simulink model "SIM_SAD_DEMO"  (R2025b)
settings: Solver=ode5  StartTime=0.0  StopTime=2*T  FixedStep=0.1  RelTol=1e-3
model workspace (MAT data in the model file):
  Pnull : Simulink.Parameter (value not decoded)
  rho_albedo_medio : Simulink.Parameter (value not decoded)
values from neighbouring files (symbols this model uses):
  Aree = zeros(10,1)    [SCRIPT_SAD_DEMO.m]
  base_seed = base_seed_MC + k    [SCRIPT_SAD_DEMO.m]
  c = astroConstants(5)*1e3    [SCRIPT_SAD_DEMO.m]
  draan = 1.99096871e-7    (= 1.99096871e-07)    [SCRIPT_SAD_DEMO.m]
  dwell_time = 30    [SCRIPT_SAD_DEMO.m]
  eps_att = deg2rad(0.2)    [SCRIPT_SAD_DEMO.m]
  eps_E = deg2rad(astroConstants(63))    [SCRIPT_SAD_DEMO.m]
  eps_h_r = 0.001    [SCRIPT_SAD_DEMO.m]
  eps_w = deg2rad(0.1)    [SCRIPT_SAD_DEMO.m]
  err_max = deg2rad(15)    [SCRIPT_SAD_DEMO.m]
  F_e = 1358    [SCRIPT_SAD_DEMO.m]
  h_r_max = 0.05    [SCRIPT_SAD_DEMO.m]
  h_r_safe = 0.001    [SCRIPT_SAD_DEMO.m]
  j_B = [0.01; 0.05; 0.01]    [SCRIPT_SAD_DEMO.m]
  J_depl = J_nom    [SCRIPT_SAD_DEMO.m]
  JD0 = juliandate(startTime)    [SCRIPT_SAD_DEMO.m]
  k_b = 200000    [SCRIPT_SAD_DEMO.m]
  Kd = K(:, 1:3)    [SCRIPT_SAD_DEMO.m]
  kep = [a,e,incl,raan,w,theta]    [SCRIPT_SAD_DEMO.m]
  Kp = K(:, 4:6)    [SCRIPT_SAD_DEMO.m]
  mu = astroConstants(13)    [SCRIPT_SAD_DEMO.m]
  n = sqrt( (mu/ (a)^3))    [SCRIPT_SAD_DEMO.m]
  n_sun = 2*pi/T_sun    (= 1.99238499086e-07)    [SCRIPT_SAD_DEMO.m]
  Nmat = [ ... (first row only)    [SCRIPT_SAD_DEMO.m]
  r_sun = 1*AU    [SCRIPT_SAD_DEMO.m]
  Re = astroConstants(23)    [SCRIPT_SAD_DEMO.m]
  rf = [ ... (first row only)    [SCRIPT_SAD_DEMO.m]
  rhod = 0.1*ones(10,1)    [SCRIPT_SAD_DEMO.m]
  rhos = zeros(10,1)    [SCRIPT_SAD_DEMO.m]
  SRP = SRP_nom    [SCRIPT_SAD_DEMO.m]
  theta = 0    [SCRIPT_SAD_DEMO.m]
  w0 = w0_nom    [SCRIPT_SAD_DEMO.m]
  w_enter = Control.w_tumbling    [SCRIPT_SAD_DEMO.m]
  w_enter_2 = Control.w_pointing    [SCRIPT_SAD_DEMO.m]
  w_exit = deg2rad(4)    [SCRIPT_SAD_DEMO.m]
  w_exit_2 = deg2rad(1.5)    [SCRIPT_SAD_DEMO.m]
symbols that are objects in the model workspace (value not decoded): Pnull, rho_albedo_medio
undefined symbols (not defined in the file or in its folder): DiscIntNeverNeededParam, Filter, Gyro, Magmeter, MTQ, q, RW, Sun_sensor
libraries: matrix_library x41, LIBRARY_SAD x40, simulink x1, cstblocks x1
(part 2 of 4)

== system SIM_SAD_DEMO/Subsystem ==
  q_e : Inport
  Constant : Constant  Value=0
  Constant1 : Constant
  Demux : Demux
  Gain : Gain  Gain=2
  Gain1 : Gain  Gain=2
  Gain2 : Gain  Gain=2
  Gain3 : Gain  Gain=-1
  Product : Product
  Relational Operator : RelationalOperator  Operator=<=  OutDataTypeStr=boolean  RndMeth=Simplest  InputSameDT=off
  Switch : Switch  Criteria=u2 > Threshold  SaturateOnIntegerOverflow=off  InputSameDT=off
  Vector Concatenate : Concatenate  NumInputs=3
  Out1 : Outport
  wires:
  Vector Concatenate/1 -> Product/1
  Demux/3 -> Gain2/1
  Gain3/1 -> Switch/3
  Gain2/1 -> Vector Concatenate/3
  Constant/1 -> Relational Operator/2
  Relational Operator/1 -> Switch/2
  Constant1/1 -> Switch/1, Gain3/1
  Gain1/1 -> Vector Concatenate/2
  Demux/4 -> Relational Operator/1
  Switch/1 -> Product/2
  Demux/1 -> Gain/1
  Demux/2 -> Gain1/1
  Gain/1 -> Vector Concatenate/1
  Product/1 -> Out1/1
  q_e/1 -> Demux/1

== system SIM_SAD_DEMO/q-->DCM ==
  note: ORTHONORMALITY ERROR A_B/N RECONSTRUCTED CHECK
  q_e : Inport
  Demux1 : Demux  Outputs=9
  Demux2 : Demux
  Display : Display
  Gain4 : Gain  Gain=2
  Gain5 : Gain  Gain=2
  I : Constant  Value=[1,0,0;0,1,0;0,0,1]
  I1 : Constant  Value=[1,0,0;0,1,0;0,0,1]
  MatrixMultiply : Product  Multiplication=Matrix(*)
  MatrixMultiply1 : Product  Multiplication=Matrix(*)
  MatrixMultiply2 : Product  Multiplication=Matrix(*)
  Product1 : Product
  Product2 : Product
  Reshape1 : Reshape  OutputDimensionality=Customize  OutputDimensions=[9,1]
  Scope1 : Scope  NumInputPorts=9
      settings: ActiveDisplayYMinimum=0.78091180257448345  ActiveDisplayYMaximum=1.0243231881597876  DataLoggingVariableName=ScopeData56
  Square : Math  Operator=square
  Sum4 : Sum  Inputs=+-
  Sum5 : Sum  Inputs=+-
  Sum6 : Sum  Inputs=-++
  To Workspace2 : ToWorkspace  VariableName=A_e  SampleTime=-1
  Transpose : Math  Operator=transpose
  Transpose2 : Math  Operator=transpose
  Vector Concatenate1 : Concatenate  NumInputs=3
  "[qΛ]" : Subsystem
  A_B/N_e : Outport
  wires:
  Demux1/2 -> Scope1/2  "A_12"
  MatrixMultiply/1 -> Sum4/2  "qTq"
  Demux2/3 -> Vector Concatenate1/3
  Gain5/1 -> Product1/2  "2q4"
  Product1/1 -> Sum6/1  "2*q4*[qΛ ]"
  Demux2/4 -> Gain5/1, Square/1  "q4"
  Demux1/6 -> Scope1/6  "A_23"
  Product2/1 -> Sum6/2  "(q4^2-qTq)*I"
  Demux2/1 -> Vector Concatenate1/1
  Gain4/1 -> Sum6/3  "2*q*qT"
  Demux1/5 -> Scope1/5  "A_22"
  I1/1 -> Sum5/2
  "[qΛ]"/1("[qΛ]") -> Product1/1
  MatrixMultiply1/1 -> Gain4/1  "qqT"
  Transpose2/1 -> MatrixMultiply2/1  "qT"
  Square/1 -> Sum4/1
  Demux1/8 -> Scope1/8  "A_32"
  Sum4/1 -> Product2/1
  Demux1/7 -> Scope1/7  "A_31"
  I/1 -> Product2/2
  Demux1/9 -> Scope1/9  "A_33"
  Vector Concatenate1/1 -> Transpose/1, MatrixMultiply1/1, MatrixMultiply/2  "q"
  Demux2/2 -> Vector Concatenate1/2
  Sum6/1 -> Transpose2/1, MatrixMultiply2/2, Reshape1/1, To Workspace2/1, A_B/N_e/1  "A_B/N"
  Demux1/1 -> Scope1/1  "A_11"
  MatrixMultiply2/1 -> Sum5/1  "qTq"
  Demux1/4 -> Scope1/4  "A_21"
  Transpose/1 -> MatrixMultiply1/2, MatrixMultiply/1  "qT"
  Reshape1/1 -> Demux1/1
  q_e/1 -> Demux2/1, "[qΛ]"/1(q), Display/1
  Demux1/3 -> Scope1/3  "A_13"

== system SIM_SAD_DEMO/q-->DCM1 ==
  note: ORTHONORMALITY ERROR A_B/N RECONSTRUCTED CHECK
  q_m : Inport
  Demux1 : Demux  Outputs=9
  Demux2 : Demux
  Display : Display
  Gain4 : Gain  Gain=2
  Gain5 : Gain  Gain=2
  I : Constant  Value=[1,0,0;0,1,0;0,0,1]
  I1 : Constant  Value=[1,0,0;0,1,0;0,0,1]
  MatrixMultiply : Product  Multiplication=Matrix(*)
  MatrixMultiply1 : Product  Multiplication=Matrix(*)
  MatrixMultiply2 : Product  Multiplication=Matrix(*)
  Product1 : Product
  Product2 : Product
  Reshape1 : Reshape  OutputDimensionality=Customize  OutputDimensions=[9,1]
  Scope1 : Scope  NumInputPorts=9
      settings: ActiveDisplayYMinimum=0.78091180257448345  ActiveDisplayYMaximum=1.0243231881597876  DataLoggingVariableName=ScopeData56
  Square : Math  Operator=square
  Sum4 : Sum  Inputs=+-
  Sum5 : Sum  Inputs=+-
  Sum6 : Sum  Inputs=-++
  Transpose : Math  Operator=transpose
  Transpose2 : Math  Operator=transpose
  Vector Concatenate1 : Concatenate  NumInputs=3
  "[qΛ]" : Subsystem
  A_B/N_m : Outport
  wires:
  Demux1/2 -> Scope1/2  "A_12"
  MatrixMultiply/1 -> Sum4/2  "qTq"
  Demux2/3 -> Vector Concatenate1/3
  Gain5/1 -> Product1/2  "2q4"
  Product1/1 -> Sum6/1  "2*q4*[qΛ ]"
  Demux2/4 -> Gain5/1, Square/1  "q4"
  Demux1/6 -> Scope1/6  "A_23"
  Product2/1 -> Sum6/2  "(q4^2-qTq)*I"
  Demux2/1 -> Vector Concatenate1/1
  Gain4/1 -> Sum6/3  "2*q*qT"
  Demux1/5 -> Scope1/5  "A_22"
  I1/1 -> Sum5/2
  "[qΛ]"/1("[qΛ]") -> Product1/1
  MatrixMultiply1/1 -> Gain4/1  "qqT"
  Transpose2/1 -> MatrixMultiply2/1  "qT"
  Square/1 -> Sum4/1
  Demux1/8 -> Scope1/8  "A_32"
  Sum4/1 -> Product2/1
  Demux1/7 -> Scope1/7  "A_31"
  I/1 -> Product2/2
  Demux1/9 -> Scope1/9  "A_33"
  Vector Concatenate1/1 -> Transpose/1, MatrixMultiply1/1, MatrixMultiply/2  "q"
  Demux2/2 -> Vector Concatenate1/2
  Sum6/1 -> Transpose2/1, MatrixMultiply2/2, Reshape1/1, A_B/N_m/1  "A_B/N"
  Demux1/1 -> Scope1/1  "A_11"
  MatrixMultiply2/1 -> Sum5/1  "qTq"
  Demux1/4 -> Scope1/4  "A_21"
  Transpose/1 -> MatrixMultiply1/2, MatrixMultiply/1  "qT"
  Reshape1/1 -> Demux1/1
  q_m/1 -> Demux2/1, "[qΛ]"/1(q), Display/1
  Demux1/3 -> Scope1/3  "A_13"

== system SIM_SAD_DEMO/ACTUATORS/Detumbling (MTQ only) ==
  note: REACTION WHEEL
  note: MAGNETORQUERS
  M_c : Inport
  B_B_m : Inport  Port=2
  h_r_feed : Inport  Port=3
  Constant : Constant  Value=0
  Constant1 : Constant  Value=RW.A
  Cross Product : matrix_library/Cross Product
  Cross Product2 : matrix_library/Cross Product
  Delay : Delay  DelayLength=1  SampleTime=q.Ts
  Demux : Demux  Outputs=3
  Discrete-Time Integrator : DiscreteIntegrator  InitialConditionSource=external  SampleTime=-1  ICPrevOutput=DiscIntNeverNeededParam  ICPrevScaledInput=DiscIntNeverNeededParam
  Divide : Product  Inputs=*/
  MatrixMultiply : Product  Multiplication=Matrix(*)
  Norm1 : Subsystem
  Saturation3 : Saturate  UpperLimit=MTQ.D_max_XY  LowerLimit=-MTQ.D_max_XY
  Saturation4 : Saturate  UpperLimit=MTQ.D_max_XY  LowerLimit=-MTQ.D_max_XY
  Saturation5 : Saturate  UpperLimit=MTQ.D_max_Z  LowerLimit=-MTQ.D_max_Z
  Scope : Scope
      settings: ActiveDisplayYMinimum=-14.411553950631344  ActiveDisplayYMaximum=16.201380468990443  DataLoggingVariableName=ScopeData111
  Scope6 : Scope
      settings: ActiveDisplayYMinimum=-2.5  ActiveDisplayYMaximum=2.5  DataLoggingVariableName=ScopeData112
  Square1 : Math  Operator=square
  Sum : Sum
  Vector Concatenate1 : Concatenate  NumInputs=3
  M_act : Outport
  h_r : Outport  Port=2
  wires:
  Cross Product2/1 -> Sum/1  "M_MTQ"
  Saturation3/1 -> Vector Concatenate1/1
  Demux/2 -> Saturation4/1
  Demux/1 -> Saturation3/1
  Saturation4/1 -> Vector Concatenate1/2
  Norm1/1(Out1) -> Square1/1
  Cross Product/1 -> Divide/1
  Square1/1 -> Divide/2
  Saturation5/1 -> Vector Concatenate1/3
  Vector Concatenate1/1 -> Cross Product2/1, Scope6/1  "D_eff"
  Divide/1 -> Scope/1, Demux/1  "D"
  Demux/3 -> Saturation5/1
  B_B_m/1 -> Cross Product2/2, Cross Product/1, Norm1/1(In1)  "B_B_m"
  M_c/1 -> Cross Product/2
  Constant/1 -> MatrixMultiply/2, Discrete-Time Integrator/1  "h_r_dot"
  Discrete-Time Integrator/1 -> h_r/1  "h_r"
  h_r_feed/1 -> Delay/1
  Sum/1 -> M_act/1
  Constant1/1 -> MatrixMultiply/1
  MatrixMultiply/1 -> Sum/2  "M_RW"
  Delay/1 -> Discrete-Time Integrator/2

== system SIM_SAD_DEMO/ACTUATORS/Norm ==
  note: square
  B_B_m : Inport
  Sqrt : Sqrt
  Square1 : Math  Operator=square
  Sum of Elements : Sum  Inputs=+
  Out1 : Outport
  wires:
  Sum of Elements/1 -> Sqrt/1
  B_B_m/1 -> Square1/1
  Sqrt/1 -> Out1/1
  Square1/1 -> Sum of Elements/1

== system SIM_SAD_DEMO/ACTUATORS/Norm1 ==
  note: square
  In1 : Inport
  Sqrt : Sqrt
  Square1 : Math  Operator=square
  Sum of Elements : Sum  Inputs=+
  Out1 : Outport
  wires:
  Sum of Elements/1 -> Sqrt/1
  In1/1 -> Square1/1
  Sqrt/1 -> Out1/1
  Square1/1 -> Sum of Elements/1

== system SIM_SAD_DEMO/ACTUATORS/RW Desaturation ==
  note: MAGNETORQUERS
  note: REACTION WHEEL (only for h_r)
  h_r_feed : Inport
  B_B_m : Inport  Port=2
  -M_max : Gain  Gain=-RW.T_max
  Constant : Constant  Value=RW.A
  Cross Product : matrix_library/Cross Product
  Delay : Delay  DelayLength=1  SampleTime=q.Ts
  Demux : Demux  Outputs=3
  Discrete-Time Integrator : DiscreteIntegrator  InitialConditionSource=external  SampleTime=-1  ICPrevOutput=DiscIntNeverNeededParam  ICPrevScaledInput=DiscIntNeverNeededParam
  Divide : Product  Inputs=*/
  M_max : Gain  Gain=RW.T_max
  MatrixMultiply : Product  Multiplication=Matrix(*)
  Saturation3 : Saturate  UpperLimit=MTQ.D_max_XY  LowerLimit=-MTQ.D_max_XY
  Saturation4 : Saturate  UpperLimit=MTQ.D_max_XY  LowerLimit=-MTQ.D_max_XY
  Saturation5 : Saturate  UpperLimit=MTQ.D_max_Z  LowerLimit=-MTQ.D_max_Z
  Scope{,1..6} (7 alike) : Scope
      Scope settings: ActiveDisplayYMinimum=-1  ActiveDisplayYMaximum=1  DataLoggingVariableName=ScopeData120
      Scope1 settings: ActiveDisplayYMinimum=-1  ActiveDisplayYMaximum=1  DataLoggingVariableName=ScopeData122
      Scope2 settings: ActiveDisplayYMinimum=-1  ActiveDisplayYMaximum=1  DataLoggingVariableName=ScopeData123
      Scope3 settings: ActiveDisplayYMinimum=-1  ActiveDisplayYMaximum=1  DataLoggingVariableName=ScopeData124
      Scope4 settings: ActiveDisplayYMinimum=-1  ActiveDisplayYMaximum=1  DataLoggingVariableName=ScopeData126
      Scope5 settings: ActiveDisplayYMinimum=-1  ActiveDisplayYMaximum=1  DataLoggingVariableName=ScopeData127
      Scope6 settings: ActiveDisplayYMinimum=-0.0068500524485620249  ActiveDisplayYMaximum=0.056316672494284674  DataLoggingVariableName=ScopeData128
  Sign : Signum
  Sign1 : Signum
  Square : Math  Operator=square
  Vector Concatenate1 : Concatenate  NumInputs=3
  vector_norm1 : LIBRARY_SAD/vector_norm  SystemSampleTime=-1  VariantActivationTime=update diagram  EmptyChoice=off  PassThrough=off  PassThroughVariantControl=(default)  EmptyChoiceVariantControl=(default)  AllowFlexibleInterface=on  Latency=0  AutoFrameSizeCalculation=off
  M_act : Outport
  h_r : Outport  Port=2
  wires:
  h_r_feed/1 -> Delay/1
  Delay/1 -> Scope6/1, Discrete-Time Integrator/2
  Sign/1 -> -M_max/1
  Discrete-Time Integrator/1 -> Sign/1, Sign1/1, Scope1/1, h_r/1  "h_r"
  B_B_m/1 -> Scope4/1, Cross Product/2, vector_norm1/1
  Sign1/1 -> M_max/1
  vector_norm1/1 -> Square/1
  M_max/1 -> MatrixMultiply/2
  Square/1 -> Divide/2
  Demux/1 -> Saturation3/1
  Divide/1 -> Demux/1  "D"
  Demux/3 -> Saturation5/1
  Saturation5/1 -> Vector Concatenate1/3
  Saturation3/1 -> Vector Concatenate1/1
  Demux/2 -> Saturation4/1
  Saturation4/1 -> Vector Concatenate1/2
  Vector Concatenate1/1 -> Cross Product/1, Scope/1  "D_eff"
  Cross Product/1 -> M_act/1, Scope3/1  "M_MTQ_desat"
  -M_max/1 -> Discrete-Time Integrator/1, Scope2/1  "T_RW=h_r_dot"
  MatrixMultiply/1 -> Scope5/1, Divide/1
  Constant/1 -> MatrixMultiply/1

== system SIM_SAD_DEMO/ACTUATORS/Slew//tracking (MTQ + RW) ==
  note: MAGNETORQUERS
  note: REACTION WHEEL
  M_c : Inport
  B_B_m : Inport  Port=2
  w_est : Inport  Port=3
  h_r_feed : Inport  Port=4
  A* (pseudo-inverse) : Subsystem
  Constant : Constant  Value=RW.A
  Constant1 : Constant  Value=RW.A
  Cross Product : matrix_library/Cross Product
  Cross Product1 : matrix_library/Cross Product
  Cross Product2 : matrix_library/Cross Product
  Delay : Delay  DelayLength=1  SampleTime=q.Ts
  Demux : Demux  Outputs=3
  Divide : Product  Inputs=*/
  Gain : Gain  Gain=-1
  Gain1 : Gain  Gain=-1
  Integrator : Integrator  InitialConditionSource=external
  MatrixMultiply : Product  Multiplication=Matrix(*)
  MatrixMultiply1 : Product  Multiplication=Matrix(*)
  MatrixMultiply2 : Product  Multiplication=Matrix(*)
  Norm1 : Subsystem
  Rate Limiter : RateLimiter  RisingSlewLimit=0.1  FallingSlewLimit=-0.1  SampleTimeMode=inherited
  Saturation : Saturate  UpperLimit=RW.T_max  LowerLimit=-RW.T_max
  Saturation3 : Saturate  UpperLimit=MTQ.D_max_XY  LowerLimit=-MTQ.D_max_XY
  Saturation4 : Saturate  UpperLimit=MTQ.D_max_XY  LowerLimit=-MTQ.D_max_XY
  Saturation5 : Saturate  UpperLimit=MTQ.D_max_Z  LowerLimit=-MTQ.D_max_Z
  Scope{,1..2,6} (4 alike) : Scope
      Scope settings: ActiveDisplayYMinimum=-14.411553950631344  ActiveDisplayYMaximum=16.201380468990443  DataLoggingVariableName=ScopeData113
      Scope1 settings: ActiveDisplayYMinimum=-0.00988821849985589  ActiveDisplayYMaximum=0.00899396649870301  DataLoggingVariableName=ScopeData116
      Scope2 settings: ActiveDisplayYMinimum=-0.000160369873046875  ActiveDisplayYMaximum=0.00015304565429687502  DataLoggingVariableName=ScopeData117
      Scope6 settings: ActiveDisplayYMinimum=-2.5  ActiveDisplayYMaximum=2.5  DataLoggingVariableName=ScopeData118
  Square1 : Math  Operator=square
  Sum : Sum  Inputs=++-
  Sum1 : Sum
  Vector Concatenate1 : Concatenate  NumInputs=3
  M_act : Outport
  h_r : Outport  Port=2
  wires:
  B_B_m/1 -> Norm1/1(In1), Cross Product/1, Cross Product2/2  "B_B_m"
  Square1/1 -> Divide/2
  Demux/1 -> Saturation3/1
  Vector Concatenate1/1 -> Cross Product2/1, Scope6/1  "D_eff"
  Saturation3/1 -> Vector Concatenate1/1
  Saturation5/1 -> Vector Concatenate1/3
  Saturation4/1 -> Vector Concatenate1/2
  Cross Product2/1 -> Sum/3, Scope2/1, Sum1/2  "M_MTQ"
  Cross Product/1 -> Divide/1
  Demux/2 -> Saturation4/1
  Norm1/1(Out1) -> Square1/1
  Demux/3 -> Saturation5/1
  Divide/1 -> Scope/1, Demux/1  "D"
  M_c/1 -> Cross Product/2, Sum/1  "M_c"
  w_est/1 -> Cross Product1/1
  MatrixMultiply/1 -> Cross Product1/2
  Constant/1 -> MatrixMultiply/1
  Cross Product1/1 -> Sum/2
  A* (pseudo-inverse)/1(A*) -> Gain/1
  Gain/1 -> MatrixMultiply1/1
  MatrixMultiply1/1 -> MatrixMultiply2/2, Rate Limiter/1  "h_r_dot"
  Rate Limiter/1 -> Integrator/1  "h_r_dot"
  h_r_feed/1 -> Delay/1
  Delay/1 -> Integrator/2
  Integrator/1 -> h_r/1, MatrixMultiply/2  "h_r"
  Constant1/1 -> MatrixMultiply2/1
  MatrixMultiply2/1 -> Gain1/1
  Gain1/1 -> Saturation/1
  Sum1/1 -> M_act/1
  Saturation/1 -> Scope1/1, Sum1/1  "M_RW"
  Sum/1 -> MatrixMultiply1/2

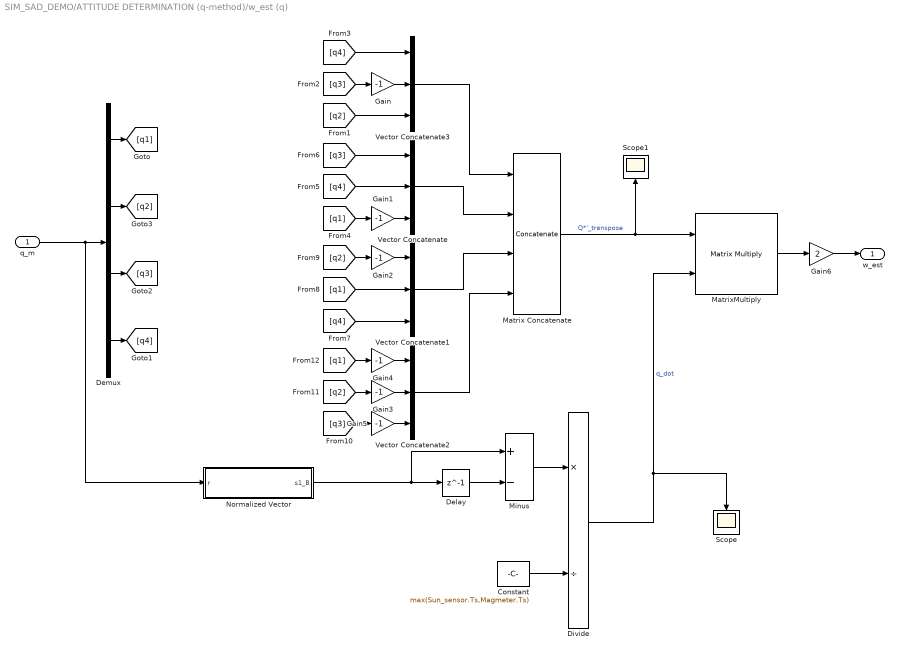
== system SIM_SAD_DEMO/ATTITUDE DETERMINATION (q-method)/w_est (q) ==
  q_m : Inport
  Constant : Constant  Value=max(Sun_sensor.Ts,Magmeter.Ts)
  Delay : Delay  DelayLength=1
  Demux : Demux
  Divide : Product  Inputs=*/
  Gain{,1..5} (6 alike) : Gain  Gain=-1
  Gain6 : Gain  Gain=2
  Matrix Concatenate : Concatenate  NumInputs=4  Mode=Multidimensional array  ConcatenateDimension=2
  MatrixMultiply : Product  Multiplication=Matrix(*)
  Minus : Sum  Inputs=+-
  Normalized Vector : Subsystem
  Scope : Scope
      settings: ActiveDisplayYMinimum=-1  ActiveDisplayYMaximum=1  DataLoggingVariableName=ScopeData67
  Scope1 : Scope
      settings: ActiveDisplayYMinimum=-1  ActiveDisplayYMaximum=1  DataLoggingVariableName=ScopeData68
  Vector Concatenate{,1..3} (4 alike) : Concatenate  NumInputs=3
  w_est : Outport
  wires:
  q_m/1 -> Normalized Vector/1(r), Demux/1
  Demux/1 -> [q1]
  Demux/2 -> [q2]
  Demux/3 -> [q3]
  Demux/4 -> [q4]
  [q4] -> Vector Concatenate3/1
  [q3] -> Gain/1
  Gain/1 -> Vector Concatenate3/2
  [q2] -> Vector Concatenate3/3
  [q1] -> Gain1/1
  [q3] -> Vector Concatenate/1
  [q4] -> Vector Concatenate1/3
  [q2] -> Gain2/1
  [q3] -> Gain5/1
  [q2] -> Gain3/1
  [q1] -> Gain4/1
  Gain3/1 -> Vector Concatenate2/2
  [q1] -> Vector Concatenate1/2
  [q4] -> Vector Concatenate/2
  Gain1/1 -> Vector Concatenate/3
  Gain2/1 -> Vector Concatenate1/1
  Gain4/1 -> Vector Concatenate2/1
  Gain5/1 -> Vector Concatenate2/3
  Vector Concatenate3/1 -> Matrix Concatenate/1
  Vector Concatenate/1 -> Matrix Concatenate/2
  Vector Concatenate1/1 -> Matrix Concatenate/3
  Vector Concatenate2/1 -> Matrix Concatenate/4
  Delay/1 -> Minus/2
  Matrix Concatenate/1 -> MatrixMultiply/1, Scope1/1  "Q*'_transpose"
  MatrixMultiply/1 -> Gain6/1
  Gain6/1 -> w_est/1
  Minus/1 -> Divide/1
  Divide/1 -> Scope/1, MatrixMultiply/2  "q_dot"
  Constant/1 -> Divide/2
  Normalized Vector/1(s1_B) -> Delay/1, Minus/1

== system SIM_SAD_DEMO/ATTITUDE TARGET (Sun Pointing)/Normalized Vector ==
  In1 : Inport
  Divide : Product  Inputs=*/
  vector_norm : LIBRARY_SAD/vector_norm  SystemSampleTime=-1  VariantActivationTime=update diagram  EmptyChoice=off  PassThrough=off  PassThroughVariantControl=(default)  EmptyChoiceVariantControl=(default)  AllowFlexibleInterface=on  Latency=0  AutoFrameSizeCalculation=off
  Out1 : Outport
  wires:
  vector_norm/1 -> Divide/2
  In1/1 -> Divide/1, vector_norm/1
  Divide/1 -> Out1/1

== system SIM_SAD_DEMO/ATTITUDE TARGET (Sun Pointing)/Normalized Vector2 ==
  r : Inport
  Divide : Product  Inputs=*/
  vector_norm : LIBRARY_SAD/vector_norm  SystemSampleTime=-1  VariantActivationTime=update diagram  EmptyChoice=off  PassThrough=off  PassThroughVariantControl=(default)  EmptyChoiceVariantControl=(default)  AllowFlexibleInterface=on  Latency=0  AutoFrameSizeCalculation=off
  s2_B : Outport
  wires:
  Divide/1 -> s2_B/1
  r/1 -> Divide/1, vector_norm/1
  vector_norm/1 -> Divide/2

== system SIM_SAD_DEMO/CONTROL/B_dot (Detumbling) ==
  w_est : Inport
  B_B_m : Inport  Port=2
  Cross Product : matrix_library/Cross Product
  Cross Product1 : matrix_library/Cross Product
  Gain : Gain  Gain=-1
  Gain1 : Gain  Gain=-k_b
  Scope{,1..3} (4 alike) : Scope
      Scope settings: ActiveDisplayYMinimum=-4.1909426960566919E-5  ActiveDisplayYMaximum=6.5793655893850854E-5  DataLoggingVariableName=ScopeData86
      Scope1 settings: ActiveDisplayYMinimum=-1  ActiveDisplayYMaximum=1  DataLoggingVariableName=ScopeData87
      Scope2 settings: ActiveDisplayYMinimum=-1  ActiveDisplayYMaximum=1  DataLoggingVariableName=ScopeData88
      Scope3 settings: ActiveDisplayYMinimum=-1  ActiveDisplayYMaximum=1  DataLoggingVariableName=ScopeData89
  M_c_detumbling : Outport
  wires:
  Cross Product1/1 -> Scope2/1, M_c_detumbling/1  "M_c_detumbling"
  Gain1/1 -> Scope3/1, Cross Product1/1  "D_req"
  Cross Product/1 -> Scope1/1, Gain1/1  "B_dot_m"
  Gain/1 -> Cross Product/1
  B_B_m/1 -> Cross Product/2, Cross Product1/2, Scope/1  "B_B_m"
  w_est/1 -> Gain/1

== system SIM_SAD_DEMO/CONTROL/ERROR VECTOR ==
  A_B/T_e : Inport
  Demux : Demux  Outputs=9
  Display : Display
  Gain : Gain  Gain=0.5
  Gain1 : Gain  Gain=0.5
  Gain2 : Gain  Gain=0.5
  Reshape : Reshape  OutputDimensionality=Customize  OutputDimensions=[9,1]
  Sum : Sum  Inputs=+-
  Sum1 : Sum  Inputs=+-
  Sum2 : Sum  Inputs=+-
  Terminator : Terminator
  Terminator1 : Terminator
  Terminator2 : Terminator
  Vector Concatenate : Concatenate  NumInputs=3
  as : Outport
  wires:
  A_B/T_e/1 -> Reshape/1
  Reshape/1 -> Demux/1
  Demux/1 -> Terminator1/1  "A_11"
  Demux/2 -> Sum2/2  "A_21"
  Demux/3 -> Sum1/1  "A_31"
  Demux/4 -> Sum2/1  "A_12"
  Demux/5 -> Terminator/1  "A_22"
  Demux/6 -> Sum/2  "A_32"
  Demux/7 -> Sum1/2  "A_13"
  Demux/8 -> Sum/1  "A_23"
  Demux/9 -> Terminator2/1  "A_33"
  Sum/1 -> Gain/1
  Sum1/1 -> Gain1/1
  Sum2/1 -> Gain2/1
  Gain/1 -> Vector Concatenate/1  "first  component"
  Gain1/1 -> Vector Concatenate/2  "second component"
  Gain2/1 -> Vector Concatenate/3  "third component"
  Vector Concatenate/1 -> as/1, Display/1

== system SIM_SAD_DEMO/CONTROL/RW Desaturation ==
  Constant : Constant  Value=0
  Constant1 : Constant  Value=0
  Constant2 : Constant  Value=0
  Vector Concatenate : Concatenate  NumInputs=3
  M_c_desat : Outport
  wires:
  Constant/1 -> Vector Concatenate/1
  Constant2/1 -> Vector Concatenate/3
  Constant1/1 -> Vector Concatenate/2
  Vector Concatenate/1 -> M_c_desat/1

== system SIM_SAD_DEMO/CONTROL/Slew Manouvre//pointing ==
  note: CONTROL LOGIC: u = -kp*as - kd*w
      | as = components of matrix A_e
  w_est : Inport
  as : Inport  Port=2
  Constant : Constant  Value=Kd
  Constant1 : Constant  Value=Kp
  Gain : Gain  Gain=-1
  Gain1 : Gain  Gain=-1
  Matrix Multiply : Product  Multiplication=Matrix(*)
  Matrix Multiply1 : Product  Multiplication=Matrix(*)
  Scope : Scope
      settings: ActiveDisplayYMinimum=-0.23306272336823153  ActiveDisplayYMaximum=0.11744428316780303  DataLoggingVariableName=ScopeData90
  Sum of Elements : Sum
  Mc_slew : Outport
  wires:
  Gain/1 -> Matrix Multiply/2
  as/1 -> Gain1/1
  Matrix Multiply/1 -> Sum of Elements/1
  Matrix Multiply1/1 -> Sum of Elements/2
  Constant1/1 -> Matrix Multiply1/1
  w_est/1 -> Gain/1
  Gain1/1 -> Matrix Multiply1/2
  Sum of Elements/1 -> Scope/1, Mc_slew/1
  Constant/1 -> Matrix Multiply/1

== system SIM_SAD_DEMO/CONTROL/Tracking ==
  note: CONTROL LOGIC: u = -kp*alpha - kd*w
      | alpha = [alpha_x; alpha_y; alpha_z] rotations under the hypothesis of small angles
  w_est : Inport
  alpha : Inport  Port=2
  Constant : Constant  Value=Kd
  Constant1 : Constant  Value=Kp
  Gain : Gain  Gain=-1
  Gain1 : Gain  Gain=-1
  Matrix Multiply : Product  Multiplication=Matrix(*)
  Matrix Multiply1 : Product  Multiplication=Matrix(*)
  Scope : Scope
      settings: ActiveDisplayYMinimum=-0.23306272336823153  ActiveDisplayYMaximum=0.11744428316780303  DataLoggingVariableName=ScopeData93
  Sum of Elements : Sum
  Mc_tracking : Outport
  wires:
  Gain1/1 -> Matrix Multiply1/2
  Gain/1 -> Matrix Multiply/2
  Sum of Elements/1 -> Scope/1, Mc_tracking/1
  w_est/1 -> Gain/1
  Matrix Multiply1/1 -> Sum of Elements/2
  Matrix Multiply/1 -> Sum of Elements/1
  Constant1/1 -> Matrix Multiply1/1
  Constant/1 -> Matrix Multiply/1
  alpha/1 -> Gain1/1

== system SIM_SAD_DEMO/DCM ---> q/q-->DCM (CHECK) ==
  note: ORTHONORMALITY ERROR A_B/N RECONSTRUCTED CHECK
  q_norm : Inport
  Demux1 : Demux  Outputs=9
  Demux2 : Demux
  Display : Display
  Gain4 : Gain  Gain=2
  Gain5 : Gain  Gain=2
  I : Constant  Value=[1,0,0;0,1,0;0,0,1]
  I1 : Constant  Value=[1,0,0;0,1,0;0,0,1]
  MatrixMultiply : Product  Multiplication=Matrix(*)
  MatrixMultiply1 : Product  Multiplication=Matrix(*)
  MatrixMultiply2 : Product  Multiplication=Matrix(*)
  Product1 : Product
  Product2 : Product
  Reshape1 : Reshape  OutputDimensionality=Customize  OutputDimensions=[9,1]
  Scope : Scope
      settings: ActiveDisplayYMinimum=-1  ActiveDisplayYMaximum=1  DataLoggingVariableName=ScopeData57
  Scope1 : Scope  NumInputPorts=9
      settings: ActiveDisplayYMinimum=-1.2499999988864972  ActiveDisplayYMaximum=1.2499999998762776  DataLoggingVariableName=ScopeData56
  Square : Math  Operator=square
  Sum4 : Sum  Inputs=+-
  Sum5 : Sum  Inputs=+-
  Sum6 : Sum  Inputs=-++
  Transpose : Math  Operator=transpose
  Transpose2 : Math  Operator=transpose
  Vector Concatenate1 : Concatenate  NumInputs=3
  "[qΛ]" : Subsystem
  wires:
  Demux1/3 -> Scope1/3  "A_13"
  q_norm/1 -> Display/1, "[qΛ]"/1(q), Demux2/1
  Reshape1/1 -> Demux1/1
  Transpose/1 -> MatrixMultiply/1, MatrixMultiply1/2  "qT"
  Demux1/4 -> Scope1/4  "A_21"
  MatrixMultiply2/1 -> Sum5/1  "qTq"
  Demux1/1 -> Scope1/1  "A_11"
  Sum6/1 -> Reshape1/1, MatrixMultiply2/2, Transpose2/1  "A_B/N"
  Demux2/2 -> Vector Concatenate1/2
  Vector Concatenate1/1 -> MatrixMultiply/2, MatrixMultiply1/1, Transpose/1  "q"
  Demux1/9 -> Scope1/9  "A_33"
  Sum5/1 -> Scope/1
  I/1 -> Product2/2
  Demux1/7 -> Scope1/7  "A_31"
  Sum4/1 -> Product2/1
  Demux1/8 -> Scope1/8  "A_32"
  Square/1 -> Sum4/1
  Transpose2/1 -> MatrixMultiply2/1  "qT"
  MatrixMultiply1/1 -> Gain4/1  "qqT"
  "[qΛ]"/1("[qΛ]") -> Product1/1
  I1/1 -> Sum5/2
  Demux1/5 -> Scope1/5  "A_22"
  Gain4/1 -> Sum6/3  "2*q*qT"
  Demux2/1 -> Vector Concatenate1/1
  Product2/1 -> Sum6/2  "(q4^2-qTq)*I"
  Demux1/6 -> Scope1/6  "A_23"
  Demux2/4 -> Square/1, Gain5/1  "q4"
  Product1/1 -> Sum6/1  "2*q4*[qΛ ]"
  Gain5/1 -> Product1/2  "2q4"
  Demux2/3 -> Vector Concatenate1/3
  MatrixMultiply/1 -> Sum4/2  "qTq"
  Demux1/2 -> Scope1/2  "A_12"

== system SIM_SAD_DEMO/DCM ---> q/vector_norm ==
  r : Inport
  Sqrt : Sqrt
  Square : Math  Operator=square
  Sum of Elements : Sum  Inputs=+
  r_norm : Outport
  wires:
  Sqrt/1 -> r_norm/1
  r/1 -> Square/1
  Sum of Elements/1 -> Sqrt/1
  Square/1 -> Sum of Elements/1

== system SIM_SAD_DEMO/DCM->q (Shepperd Algorithm)/Normalized Vector1 ==
  r : Inport
  Constant : Constant  Value=1e-12
  Divide : Product  Inputs=*/
  Max : MinMax  Function=max  Inputs=2
  vector_norm : LIBRARY_SAD/vector_norm  SystemSampleTime=-1  VariantActivationTime=update diagram  EmptyChoice=off  PassThrough=off  PassThroughVariantControl=(default)  EmptyChoiceVariantControl=(default)  AllowFlexibleInterface=on  Latency=0  AutoFrameSizeCalculation=off
  r_norm : Outport
  wires:
  vector_norm/1 -> Max/1
  r/1 -> Divide/1, vector_norm/1
  Divide/1 -> r_norm/1
  Constant/1 -> Max/2
  Max/1 -> Divide/2

== system SIM_SAD_DEMO/DKE/ALBEDO_TORQUE ==
  note: Solar Radiation Pression Torque
  note: creo un blocco for each che mi permette di eseguire passo a passo ogni singola operazione del prodotto vettoriale, andando poi a crearmi il vettore uscita finale. In input ho un 10x3, però dentro il for each lavoro con delle 3x1 per semplicità, con vettori colonna quindi
  note: scarto i valori negativi perchè significa che mi trovo dalla parte opposta della faccia colpita dal sole, quindi non genero albedo, in quel caso tutto il satellite non viene colpito, quindi non mi serve creare una mask, ma basta semplicemente considerare il vettore nullo
  sun direction inertial : Inport
  Ab_n : Inport  Port=2
  S/C direction : Inport  Port=3
  Constant : Constant  Value=0
  Constant16 : Constant  Value=rf
  Constant2 : Constant  Value=Pnull
  Dot Product : DotProduct  OutDataTypeStr=Inherit: Inherit via internal rule
  For Each Subsystem1 : Subsystem  TreatAsAtomicUnit=on
  Matrix Multiply4 : Product  Multiplication=Matrix(*)
  Max : MinMax  Function=max  Inputs=2
  Normalization : Subsystem
  "Normalization " : Subsystem
  Normalization1 : Subsystem
  Reshape2 : Reshape  OutputDimensionality=Customize  OutputDimensions=[10 3]
  Ricavo i vettori forza1 : Subsystem
  Scope10 : Scope
      settings: ActiveDisplayYMinimum=-8805.2567998384475  ActiveDisplayYMaximum=8127.929464306656  DataLoggingVariableName=ScopeData17
  Scope9 : Scope
      settings: ActiveDisplayYMinimum=-9.2718061255302776E-25  ActiveDisplayYMaximum=2.6543612251060555E-24  DataLoggingVariableName=ScopeData25
  Sum of Elements2 : Sum  Inputs=+  CollapseMode=Specified dimension
  Switch : Switch  Criteria=u2 > Threshold  SaturateOnIntegerOverflow=off  InputSameDT=off
  To Workspace : ToWorkspace  VariableName=AlbRtorque  SampleTime=-1
  Transpose : Math  Operator=transpose
  Albedo_torque : Outport
  wires:
  Sum of Elements2/1 -> Transpose/1, To Workspace/1, Scope9/1
  Matrix Multiply4/1 -> Ricavo i vettori forza1/3(R_B), Normalization/1(In1)
  Normalization1/1(Out1) -> Dot Product/2
  Ricavo i vettori forza1/1(Out1) -> For Each Subsystem1/2(In2)
  For Each Subsystem1/1(Out1) -> Reshape2/1
  S/C direction/1 -> Scope10/1, Matrix Multiply4/2, Normalization1/1(R_N)
  "Normalization "/1(Out1) -> Dot Product/1
  Constant16/1 -> For Each Subsystem1/1(In1)
  Normalization/1(Out1) -> Ricavo i vettori forza1/1(" R_ B direction normalized")
  Dot Product/1 -> Max/1  "Illuminated"
  Ab_n/1 -> Matrix Multiply4/1
  sun direction inertial/1 -> "Normalization "/1(In1)
  Constant2/1 -> Switch/3
  Reshape2/1 -> Sum of Elements2/1
  Constant/1 -> Max/2
  Transpose/1 -> Switch/1
  Switch/1 -> Albedo_torque/1
  Max/1 -> Ricavo i vettori forza1/2(In2), [Illum]  "Illuminated"
  [Illum] -> Switch/2

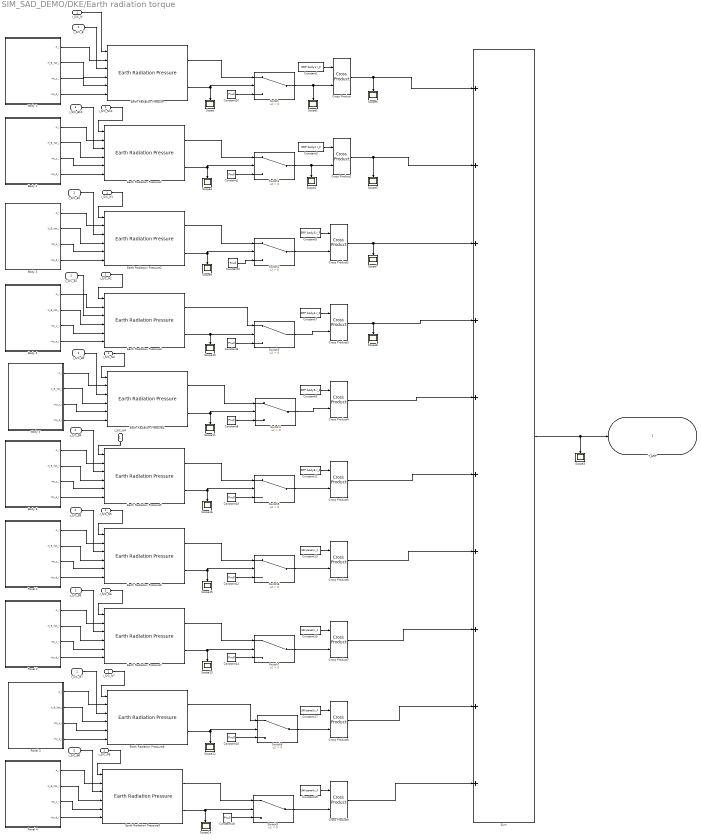
== system SIM_SAD_DEMO/DKE/Earth radiation torque ==
  r_S/C_N : Inport
  r_S/C_B : Inport  Port=2
  Body 1 : Subsystem
  Body 2 : Subsystem
  Body 3 : Subsystem
  Body 4 : Subsystem
  Body 5 : Subsystem
  Body 6 : Subsystem
  Constant1 : Constant  Value=SRP.body1.r_F
  Constant{2,4,6,8,10,12,14,16,18,20} (10 alike) : Constant  Value=Pnull
  Constant11 : Constant  Value=SRP.body6.r_F
  Constant13 : Constant  Value=SRP.panel1.r_F
  Constant15 : Constant  Value=SRP.panel2.r_F
  Constant17 : Constant  Value=SRP.panel3.r_F
  Constant19 : Constant  Value=SRP.panel4.r_F
  Constant3 : Constant  Value=SRP.body2.r_F
  Constant5 : Constant  Value=SRP.body3.r_F
  Constant7 : Constant  Value=SRP.body4.r_F
  Constant9 : Constant  Value=SRP.body5.r_F
  Cross Product{,1..9} (10 alike) : matrix_library/Cross Product
  Earth Radiation Pressure{,1..9} (10 alike) : LIBRARY_SAD/Earth Radiation Pressure  SystemSampleTime=-1  VariantActivationTime=update diagram  EmptyChoice=off  PassThrough=off  PassThroughVariantControl=(default)  EmptyChoiceVariantControl=(default)  AllowFlexibleInterface=on  Latency=0  AutoFrameSizeCalculation=off
  Panel 1 : Subsystem
  Panel 2 : Subsystem
  Panel 3 : Subsystem
  Panel 4 : Subsystem
  Scope{,1..16} (17 alike) : Scope
      Scope settings: ActiveDisplayYMinimum=-1  ActiveDisplayYMaximum=1  DataLoggingVariableName=ScopeData28
      Scope1 settings: ActiveDisplayYMinimum=-1  ActiveDisplayYMaximum=1  DataLoggingVariableName=ScopeData29
      Scope10 settings: DataLoggingVariableName=ScopeData11
      Scope11 settings: DataLoggingVariableName=ScopeData12
      Scope12 settings: DataLoggingVariableName=ScopeData13
      Scope13 settings: DataLoggingVariableName=ScopeData14
      Scope14 settings: DataLoggingVariableName=ScopeData15
      Scope15 settings: DataLoggingVariableName=ScopeData17
      Scope16 settings: DataLoggingVariableName=ScopeData18
      Scope2 settings: ActiveDisplayYMinimum=-1  ActiveDisplayYMaximum=1  DataLoggingVariableName=ScopeData30
      Scope3 settings: ActiveDisplayYMinimum=-5.1359030627651383E-25  ActiveDisplayYMaximum=9.2718061255302776E-25  DataLoggingVariableName=ScopeData31
      Scope4 settings: ActiveDisplayYMinimum=-1  ActiveDisplayYMaximum=1  DataLoggingVariableName=ScopeData32
      Scope5 settings: ActiveDisplayYMinimum=-1  ActiveDisplayYMaximum=1  DataLoggingVariableName=ScopeData33
      Scope6 settings: ActiveDisplayYMinimum=-1  ActiveDisplayYMaximum=1  DataLoggingVariableName=ScopeData34
      Scope7 settings: ActiveDisplayYMinimum=-1  ActiveDisplayYMaximum=1  DataLoggingVariableName=ScopeData35
      Scope8 settings: ActiveDisplayYMinimum=-1  ActiveDisplayYMaximum=1  DataLoggingVariableName=ScopeData36
      Scope9 settings: DataLoggingVariableName=ScopeData10
  Sum : Sum  Inputs=++++++++++
  Switch{,1..9} (10 alike) : Switch  Criteria=u2 > Threshold  SaturateOnIntegerOverflow=off  InputSameDT=off
  r_S/C_B{1..8,10} (9 alike) : InportShadow  Port=2
  r_S/C_N{1..8,10} (9 alike) : InportShadow
  T_ERP : Outport
  wires:
  Constant15/1 -> Cross Product7/1
  Switch6/1 -> Cross Product6/2
  Body 1/3(rho_s_i) -> Earth Radiation Pressure/5
  Constant6/1 -> Switch3/3
  Switch9/1 -> Cross Product9/2
  Constant13/1 -> Cross Product6/1
  Constant19/1 -> Cross Product9/1
  Cross Product4/1 -> Sum/5
  Constant16/1 -> Switch8/3
  Sum/1 -> Scope3/1, T_ERP/1
  Constant17/1 -> Cross Product8/1
  Constant1/1 -> Cross Product/1
  Switch5/1 -> Cross Product5/2
  r_S/C_B/1 -> Earth Radiation Pressure/3
  Switch3/1 -> Cross Product3/2
  Switch/1 -> Scope1/1, Cross Product/2
  Earth Radiation Pressure/2 -> Switch/2, Scope/1
  Cross Product9/1 -> Sum/10
  Cross Product3/1 -> Scope8/1, Sum/4
  Switch1/1 -> Scope2/1, Cross Product1/2
  Switch8/1 -> Cross Product8/2
  Cross Product2/1 -> Scope7/1, Sum/3
  Constant20/1 -> Switch/3
  Constant11/1 -> Cross Product5/1
  Constant8/1 -> Switch4/3
  Constant9/1 -> Cross Product4/1
  Earth Radiation Pressure/1 -> Switch/1
  Constant10/1 -> Switch5/3
  Switch4/1 -> Cross Product4/2
  Body 1/4(rho_d_i) -> Earth Radiation Pressure/6
  Cross Product5/1 -> Sum/6
  Constant3/1 -> Cross Product1/1
  Constant18/1 -> Switch9/3
  Constant14/1 -> Switch7/3
  Cross Product1/1 -> Sum/2, Scope5/1
  Constant2/1 -> Switch1/3
  Constant5/1 -> Cross Product2/1
  Constant12/1 -> Switch6/3
  Body 1/2(N_B_hat_i) -> Earth Radiation Pressure/4
  Cross Product6/1 -> Sum/7
  Body 1/1(A_i) -> Earth Radiation Pressure/2
  Cross Product7/1 -> Sum/8
  Switch2/1 -> Cross Product2/2
  Constant4/1 -> Switch2/3
  Switch7/1 -> Cross Product7/2
  Cross Product8/1 -> Sum/9
  Constant7/1 -> Cross Product3/1
  Cross Product/1 -> Scope6/1, Sum/1
  r_S/C_N/1 -> Earth Radiation Pressure/1
  Body 2/3(rho_s_i) -> Earth Radiation Pressure1/5
  Body 2/4(rho_d_i) -> Earth Radiation Pressure1/6
  Body 2/2(N_B_hat_i) -> Earth Radiation Pressure1/4
  r_S/C_B10/1 -> Earth Radiation Pressure1/3
  r_S/C_N10/1 -> Earth Radiation Pressure1/1
  Earth Radiation Pressure1/1 -> Switch1/1
  Earth Radiation Pressure1/2 -> Scope4/1, Switch1/2
  Body 2/1(A_i) -> Earth Radiation Pressure1/2
  Earth Radiation Pressure2/1 -> Switch2/1
  Body 3/2(N_B_hat_i) -> Earth Radiation Pressure2/4
  Body 3/4(rho_d_i) -> Earth Radiation Pressure2/6
  Body 3/1(A_i) -> Earth Radiation Pressure2/2
  Earth Radiation Pressure2/2 -> Scope9/1, Switch2/2
  r_S/C_N1/1 -> Earth Radiation Pressure2/1
  r_S/C_B1/1 -> Earth Radiation Pressure2/3
  Body 3/3(rho_s_i) -> Earth Radiation Pressure2/5
  Earth Radiation Pressure3/1 -> Switch3/1
  Body 4/2(N_B_hat_i) -> Earth Radiation Pressure3/4
  Body 4/4(rho_d_i) -> Earth Radiation Pressure3/6
  Body 4/1(A_i) -> Earth Radiation Pressure3/2
  Earth Radiation Pressure3/2 -> Switch3/2, Scope10/1
  r_S/C_N2/1 -> Earth Radiation Pressure3/1
  r_S/C_B2/1 -> Earth Radiation Pressure3/3
  Body 4/3(rho_s_i) -> Earth Radiation Pressure3/5
  Earth Radiation Pressure4/1 -> Switch4/1
  Body 5/2(N_B_hat_i) -> Earth Radiation Pressure4/4
  Body 5/4(rho_d_i) -> Earth Radiation Pressure4/6
  Body 5/1(A_i) -> Earth Radiation Pressure4/2
  Earth Radiation Pressure4/2 -> Scope11/1, Switch4/2
  r_S/C_N3/1 -> Earth Radiation Pressure4/1
  r_S/C_B3/1 -> Earth Radiation Pressure4/3
  Body 5/3(rho_s_i) -> Earth Radiation Pressure4/5
  Earth Radiation Pressure5/1 -> Switch5/1
  Body 6/2(N_B_hat_i) -> Earth Radiation Pressure5/4
  Body 6/4(rho_d_i) -> Earth Radiation Pressure5/6
  Body 6/1(A_i) -> Earth Radiation Pressure5/2
  Earth Radiation Pressure5/2 -> Scope16/1, Switch5/2
  r_S/C_N4/1 -> Earth Radiation Pressure5/1
  r_S/C_B4/1 -> Earth Radiation Pressure5/3
  Body 6/3(rho_s_i) -> Earth Radiation Pressure5/5
  Earth Radiation Pressure6/1 -> Switch6/1
  Panel 1/2(N_B_hat_i) -> Earth Radiation Pressure6/4
  Panel 1/4(rho_d_i) -> Earth Radiation Pressure6/6
  Panel 1/1(A_i) -> Earth Radiation Pressure6/2
  Earth Radiation Pressure6/2 -> Scope15/1, Switch6/2
  r_S/C_N5/1 -> Earth Radiation Pressure6/1
  r_S/C_B5/1 -> Earth Radiation Pressure6/3
  Panel 1/3(rho_s_i) -> Earth Radiation Pressure6/5
  Earth Radiation Pressure7/1 -> Switch7/1
  Panel 2/2(N_B_hat_i) -> Earth Radiation Pressure7/4
  Panel 2/4(rho_d_i) -> Earth Radiation Pressure7/6
  Panel 2/1(A_i) -> Earth Radiation Pressure7/2
  Earth Radiation Pressure7/2 -> Scope13/1, Switch7/2
  r_S/C_N6/1 -> Earth Radiation Pressure7/1
  r_S/C_B6/1 -> Earth Radiation Pressure7/3
  Panel 2/3(rho_s_i) -> Earth Radiation Pressure7/5
  Earth Radiation Pressure8/1 -> Switch8/1
  Panel 3/2(N_B_hat_i) -> Earth Radiation Pressure8/4
  Panel 3/4(rho_d_i) -> Earth Radiation Pressure8/6
  Panel 3/1(A_i) -> Earth Radiation Pressure8/2
  Earth Radiation Pressure8/2 -> Scope12/1, Switch8/2
  r_S/C_N7/1 -> Earth Radiation Pressure8/1
  r_S/C_B7/1 -> Earth Radiation Pressure8/3
  Panel 3/3(rho_s_i) -> Earth Radiation Pressure8/5
  Earth Radiation Pressure9/1 -> Switch9/1
  Panel 4/2(N_B_hat_i) -> Earth Radiation Pressure9/4
  Panel 4/4(rho_d_i) -> Earth Radiation Pressure9/6
  Panel 4/1(A_i) -> Earth Radiation Pressure9/2
  Earth Radiation Pressure9/2 -> Scope14/1, Switch9/2
  r_S/C_N8/1 -> Earth Radiation Pressure9/1
  r_S/C_B8/1 -> Earth Radiation Pressure9/3
  Panel 4/3(rho_s_i) -> Earth Radiation Pressure9/5

== system SIM_SAD_DEMO/DKE/Earth-S//C Orbit ==
  Keplerian Elements : Inport
  n : Inport  Port=2
  Conic Equation : Subsystem
  Constant1 : Constant
  Constant2 : Constant  Value=2
  Constant3 : Constant  Value=2
  Constant4 : Constant
  Constant5 : Constant  Value=3/2
  Cos : Trigonometry  Operator=cos
  Demux : Demux  Outputs=6
      settings: DisplayOption=none
  Divide1 : Product  Inputs=**/
  Gain{1..4} (4 alike) : Gain  Gain=pi/180
  Integrator : Integrator  InitialConditionSource=external  InitialCondition=theta  WrapState=on  WrappedStateUpperValue=2*pi  WrappedStateLowerValue=0
  Power : Math  Operator=pow
  Power1 : Math  Operator=pow
  Power2 : Math  Operator=pow
  Product1 : Product
  Sum : Sum
  Sum1 : Sum  Inputs=+-
  Sun-synchronous Orbit : Integrator  InitialConditionSource=external  WrapState=on  WrappedStateUpperValue=2*pi  WrappedStateLowerValue=0
  dRAAN_dt : Constant  Value=draan
  r (Inertial Frame) : Subsystem
  r_S/C_N : Outport
  theta_rad(t) : Outport  Port=2
  incl_rad : Outport  Port=3
  theta_dot : Outport  Port=4
  wires:
  Keplerian Elements/1 -> Demux/1
  Demux/1 -> Conic Equation/1(a)  "a"
  Demux/2 -> Product1/1, Power1/1, Conic Equation/2(e)  "e"
  Demux/3 -> Gain3/1  "incl"
  Demux/4 -> Gain2/1  "raan"
  Demux/5 -> Gain1/1  "w"
  Demux/6 -> Gain4/1  "theta"
  Constant1/1 -> Sum/1
  Cos/1 -> Product1/2
  Product1/1 -> Sum/2
  Sum/1 -> Power/1
  Constant2/1 -> Power/2
  Power/1 -> Divide1/2
  Constant3/1 -> Power1/2
  Power1/1 -> Sum1/2
  Constant4/1 -> Sum1/1
  Constant5/1 -> Power2/2
  Sum1/1 -> Power2/1
  Power2/1 -> Divide1/3
  Gain3/1 -> r (Inertial Frame)/3(incl_rad), incl_rad/1  "incl_rad"
  Gain2/1 -> Sun-synchronous Orbit/2  "raan_rad"
  Gain1/1 -> r (Inertial Frame)/5(w_rad)  "w_rad"
  r (Inertial Frame)/1(r_N) -> r_S/C_N/1
  n/1 -> Divide1/1
  Gain4/1 -> Integrator/2  "theta_rad"
  Conic Equation/1(r) -> r (Inertial Frame)/1(r)
  Integrator/1 -> Conic Equation/3(theta_rad(t)), theta_rad(t)/1, r (Inertial Frame)/2(theta_rad(t)), Cos/1  "theta_rad(t)"
  Divide1/1 -> Integrator/1, theta_dot/1  "theta_dot"
  dRAAN_dt/1 -> Sun-synchronous Orbit/1
  Sun-synchronous Orbit/1 -> r (Inertial Frame)/4(raan_rad)  "raan_rad"

== system SIM_SAD_DEMO/DKE/Euler Equations (vectorial) ==
  I_matrix : Inport
  T : Inport  Port=2
  Cross Product : matrix_library/Cross Product
  Integrator : Integrator  InitialCondition=w0
  Matrix Divide : Product  Inputs=/  Multiplication=Matrix(*)
  MatrixMultiply : Product  Multiplication=Matrix(*)
  Product : Product  Multiplication=Matrix(*)
  Sum : Sum  Inputs=+-
  w_B : Outport
  wires:
  Matrix Divide/1 -> Product/1  "(I_matrix)^-1"
  I_matrix/1 -> MatrixMultiply/1, Matrix Divide/1  "I_matrix"
  Integrator/1 -> Cross Product/1, MatrixMultiply/2, w_B/1  "w"
  Product/1 -> Integrator/1  "w_dot"
  T/1 -> Sum/1
  Cross Product/1 -> Sum/2
  MatrixMultiply/1 -> Cross Product/2
  Sum/1 -> Product/2

== system SIM_SAD_DEMO/DKE/Gravity Gradient Torque ==
  I_matrix : Inport
  r_S/C_B : Inport  Port=2
  c_B : Inport  Port=3
  Constant : Constant  Value=3
  Constant1 : Constant  Value=mu
  Constant4 : Constant  Value=3
  Cross Product : matrix_library/Cross Product
  Divide : Product  Inputs=**/*
  MatrixMultiply : Product  Multiplication=Matrix(*)
  Power : Math  Operator=pow
  Scope : Scope
      settings: ActiveDisplayYMinimum=-1  ActiveDisplayYMaximum=1  DataLoggingVariableName=ScopeData99
  vector_norm : LIBRARY_SAD/vector_norm  SystemSampleTime=-1  VariantActivationTime=update diagram  EmptyChoice=off  PassThrough=off  PassThroughVariantControl=(default)  EmptyChoiceVariantControl=(default)  AllowFlexibleInterface=on  Latency=0  AutoFrameSizeCalculation=off
  T_GG : Outport
  wires:
  r_S/C_B/1 -> vector_norm/1
  Constant4/1 -> Power/2
  Constant/1 -> Divide/1
  Constant1/1 -> Divide/2
  Power/1 -> Divide/3
  I_matrix/1 -> MatrixMultiply/1
  c_B/1 -> MatrixMultiply/2, Cross Product/1
  MatrixMultiply/1 -> Cross Product/2
  Cross Product/1 -> Divide/4
  Divide/1 -> T_GG/1
  vector_norm/1 -> Scope/1, Power/1

== system SIM_SAD_DEMO/DKE/Kinematics (DCM) ==
  A_LVLH/N : Inport
  w_x : Inport  Port=2
  w_y : Inport  Port=3
  w_z : Inport  Port=4
  DCM Orthonormalisation : LIBRARY_SAD/DCM Orthonormalisation  SystemSampleTime=-1  VariantActivationTime=update diagram  EmptyChoice=off  PassThrough=off  PassThroughVariantControl=(default)  EmptyChoiceVariantControl=(default)  AllowFlexibleInterface=on  Latency=0  AutoFrameSizeCalculation=off
  DCM w matrix : LIBRARY_SAD/DCM w matrix  SystemSampleTime=-1  VariantActivationTime=update diagram  EmptyChoice=off  PassThrough=off  PassThroughVariantControl=(default)  EmptyChoiceVariantControl=(default)  AllowFlexibleInterface=on  Latency=0  AutoFrameSizeCalculation=off
  Gain : Gain  Gain=-1
  Integrator : Integrator  InitialConditionSource=external
  Product : Product  Multiplication=Matrix(*)
  To Workspace : ToWorkspace  VariableName=A_B_N  SampleTime=-1
  To Workspace1 : ToWorkspace  VariableName=A_B_N_ortho  SampleTime=-1
  A_B/N : Outport
  wires:
  A_LVLH/N/1 -> Integrator/2
  w_y/1 -> DCM w matrix/2
  w_z/1 -> DCM w matrix/3
  Integrator/1 -> To Workspace/1, DCM Orthonormalisation/1  "A_B/N"
  Product/1 -> Integrator/1  "A_dot"
  DCM w matrix/1 -> Gain/1
  w_x/1 -> DCM w matrix/1
  Gain/1 -> Product/1
  DCM Orthonormalisation/1 -> To Workspace1/1, A_B/N/1, Product/2  "A_B/N"

== system SIM_SAD_DEMO/DKE/Magnetic Torque ==
  A_B/N : Inport
  r_S/C_N : Inport  Port=2
  B_N (IGRF Model - Order N) : LIBRARY_SAD/B_N (IGRF Model - Order N)  SystemSampleTime=-1  VariantActivationTime=update diagram  EmptyChoice=off  PassThrough=off  PassThroughVariantControl=(default)  EmptyChoiceVariantControl=(default)  AllowFlexibleInterface=on  Latency=0  AutoFrameSizeCalculation=off
  Constant : Constant  Value=j_B
  Cross Product : matrix_library/Cross Product
  Display : Display
  IGRF magnetic torque : Subsystem
  MatrixMultiply : Product  Multiplication=Matrix(*)
  Scope : Scope
      settings: ActiveDisplayYMinimum=-1  ActiveDisplayYMaximum=1  DataLoggingVariableName=ScopeData5
  Scope1 : Scope
      settings: ActiveDisplayYMinimum=-1  ActiveDisplayYMaximum=1  DataLoggingVariableName=ScopeData22
  Scope13 : Scope
      settings: ActiveDisplayYMinimum=-1  ActiveDisplayYMaximum=1  DataLoggingVariableName=ScopeData37
  T_M : Outport
  B_N : Outport  Port=2
  B_B : Outport  Port=3
  wires:
  r_S/C_N/1 -> IGRF magnetic torque/1(r_S/C_N), B_N (IGRF Model - Order N)/1, Display/1
  A_B/N/1 -> MatrixMultiply/1
  MatrixMultiply/1 -> B_B/1, Scope/1, Cross Product/2  "B_B"
  Constant/1 -> Cross Product/1
  Cross Product/1 -> T_M/1
  B_N (IGRF Model - Order N)/1 -> B_N/1, MatrixMultiply/2, Scope1/1
  IGRF magnetic torque/1(B_ECI) -> Scope13/1
